simulink model "rear_differencial_dense_1"  (R2022b)
settings: Solver=FixedStepDiscrete  StartTime=0.0  StopTime=10.0  FixedStep=0.001  RelTol=1e-3  EnableMultiTasking=on
PreLoadFcn:
  | PowerOn_data
InitFcn:
  | EcoCoder_PreCheckLic();
values from neighbouring files (symbols this model uses):
  Accelerate_Percent_BreakPoints = uint8([0  2  5  10  20  30  40  50  60  70  80  90  100])    [PowerOn_data.m]
  MotorSpeed_BreakPoints = uint16(linspace(0,18000,13))    [PowerOn_data.m]
  Torque_Table = int8([ ... (first row only)    [PowerOn_data.m]
undefined symbols (not defined in the file or in its folder): HV_Botton, Inverter_Button, SC_Closed
libraries: CoderSF_BSW_Libs x83, SF_CanService_Libs x17, CoderSF_ADC2Volt_Libs x5, simulink x2, dspswit3 x1
(part 2 of 2)

== system rear_differencial_dense_1/CAN/CAN Read/SAS__CAN ==
  Bus Creator : BusCreator  Inputs=2
  Bus Creator1 : BusCreator  Inputs=7
  Read CAN Message : SF_CanService_Libs/Read CAN Message  typeCAN=Connected  channel=CAN_A  mEn=off  msgInfo=steering_angle_sensor  msgItermStore=Steering_Wheel_Angle  msgIterm=Steering_Wheel_Angle  valid=on  stale=on  motoBit=off  setSignalName=on  flgCustomMonitorVariableRules=on  defineSignalName=off  prefixSignal=''  flgValTest=off  flgNoFixed=on  tSample=Task_Inherit  modeCode=Parameterless
  Terminator : Terminator
  tag scope: SAS=global
  wires:
  Read CAN Message/7 -> Bus Creator1/5  "Function_SafetyRelated"
  Bus Creator1/1 -> [SAS]
  Read CAN Message/1 -> Bus Creator/1
  Read CAN Message/9 -> Bus Creator1/7  "SAS_SteeringAngle"
  Read CAN Message/6 -> Bus Creator1/4  "Not_Used"
  Read CAN Message/2 -> Bus Creator/2
  Read CAN Message/3 -> Bus Creator1/1  "SAS_CheckSum"
  Bus Creator/1 -> Terminator/1
  Read CAN Message/4 -> Bus Creator1/2  "Not_Used2"
  Read CAN Message/5 -> Bus Creator1/3  "SAS_MessageCounter"
  Read CAN Message/8 -> Bus Creator1/6  "SAS_SteeringAngle_Velocity"

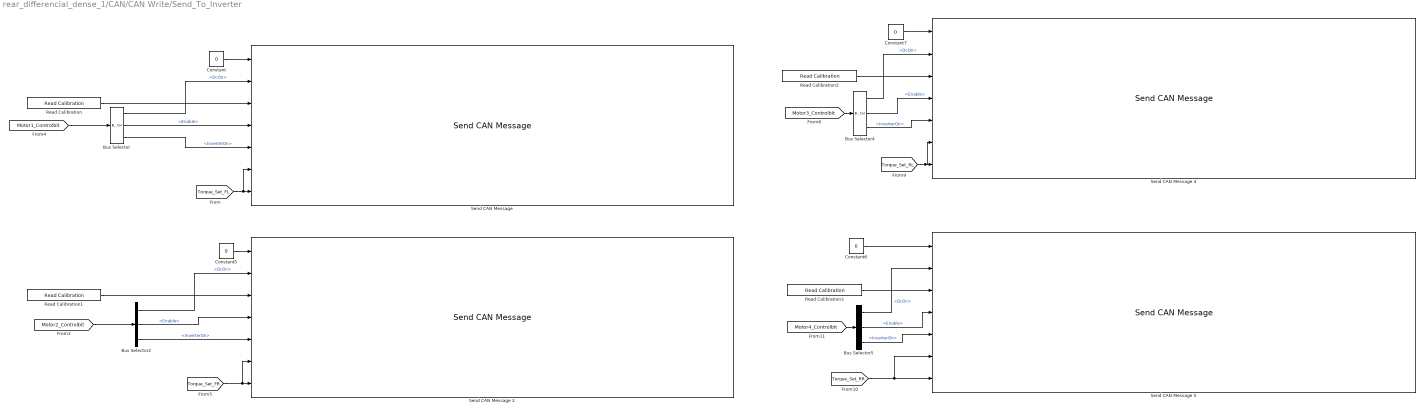
== system rear_differencial_dense_1/CAN/CAN Write/Send_To_Inverter ==
  Bus Selector{,2,4..5} (4 alike) : BusSelector  OutputSignals=DcOn,Enable,InverterOn
  Constant{,5..7} (4 alike) : Constant  Value=0  OutDataTypeStr=Inherit: Inherit via back propagation
  Read Calibration{,1..3} (4 alike) : CoderSF_BSW_Libs/Calibration & Measurement/Read Calibration  variable_name=errorset  variable_value=0  variable_type=boolean  variable_min=[]  variable_max=[]  unitStr=""  descStr=""
      settings: AttributesFormatString=value:%<variable_value> type:%<variable_type> max:%<variable_max> Min:%<variable_min>
  "Send CAN Message " : SF_CanService_Libs/Send CAN Message   typeCAN=Connected  channel=CAN_C  mEn=off  msgInfo=AMK_VCU_CAN_TorqueMode_factor_edited  msgItermStore=VCU1_0x184  msgIterm=VCU1_0x184  motoBit=off  flgNoFixed=on  tSample=Task_Inherit  modeCode=Parameterless  modeRound=Zero
  Send CAN Message 2 : SF_CanService_Libs/Send CAN Message   typeCAN=Connected  channel=CAN_C  mEn=off  msgInfo=AMK_VCU_CAN_TorqueMode_factor_edited  msgItermStore=VCU2_0x185  msgIterm=VCU2_0x185  motoBit=off  flgNoFixed=on  tSample=Task_Inherit  modeCode=Parameterless  modeRound=Zero
  Send CAN Message 4 : SF_CanService_Libs/Send CAN Message   typeCAN=Connected  channel=CAN_D  mEn=off  msgInfo=AMK_VCU_CAN_TorqueMode_factor_edited  msgItermStore=VCU3_0x188  msgIterm=VCU3_0x188  motoBit=off  flgNoFixed=on  tSample=Task_Inherit  modeCode=Parameterless  modeRound=Zero
  Send CAN Message 5 : SF_CanService_Libs/Send CAN Message   typeCAN=Connected  channel=CAN_D  mEn=off  msgInfo=AMK_VCU_CAN_TorqueMode_factor_edited  msgItermStore=VCU4_0x189  msgIterm=VCU4_0x189  motoBit=off  flgNoFixed=on  tSample=Task_Inherit  modeCode=Parameterless  modeRound=Zero
  wires:
  [Motor2_Controlbit] -> Bus Selector2/1
  Bus Selector4/2 -> Send CAN Message 4/4  "<Enable>"
  [Torque_Set_FL] -> "Send CAN Message "/6, "Send CAN Message "/7
  [Motor1_Controlbit] -> Bus Selector/1
  Read Calibration1/1 -> Send CAN Message 2/3
  Bus Selector/1 -> "Send CAN Message "/2  "<DcOn>"
  Bus Selector4/3 -> Send CAN Message 4/5  "<InverterOn>"
  [Motor3_Controlbit] -> Bus Selector4/1
  Bus Selector2/3 -> Send CAN Message 2/5  "<InverterOn>"
  Read Calibration2/1 -> Send CAN Message 4/3
  Bus Selector5/1 -> Send CAN Message 5/2  "<DcOn>"
  Bus Selector5/3 -> Send CAN Message 5/5  "<InverterOn>"
  Constant7/1 -> Send CAN Message 4/1
  [Motor4_Controlbit] -> Bus Selector5/1
  Constant5/1 -> Send CAN Message 2/1
  Bus Selector/2 -> "Send CAN Message "/4  "<Enable>"
  Read Calibration/1 -> "Send CAN Message "/3
  Bus Selector4/1 -> Send CAN Message 4/2  "<DcOn>"
  Constant/1 -> "Send CAN Message "/1
  Bus Selector5/2 -> Send CAN Message 5/4  "<Enable>"
  Read Calibration3/1 -> Send CAN Message 5/3
  Bus Selector2/1 -> Send CAN Message 2/2  "<DcOn>"
  [Torque_Set_FR] -> Send CAN Message 2/6, Send CAN Message 2/7
  Bus Selector/3 -> "Send CAN Message "/5  "<InverterOn>"
  [Torque_Set_RL] -> Send CAN Message 4/6, Send CAN Message 4/7
  Bus Selector2/2 -> Send CAN Message 2/4  "<Enable>"
  [Torque_Set_RR] -> Send CAN Message 5/6, Send CAN Message 5/7
  Constant6/1 -> Send CAN Message 5/1

== system rear_differencial_dense_1/CAN/CAN Write/Send_To_Recorder ==
  Bus Selector : BusSelector  OutputSignals=rxMCU_ActualTorque
  Bus Selector1 : BusSelector  OutputSignals=rxMCU_ActualTorque
  Bus Selector2 : BusSelector  OutputSignals=BatCurrent
  "Send CAN Message " : SF_CanService_Libs/Send CAN Message   typeCAN=Connected  channel=CAN_A  mEn=off  msgInfo=To_Recorder  msgItermStore=To_Recorder  msgIterm=To_Recorder  motoBit=off  flgNoFixed=on  tSample=Task_Inherit  modeCode=Parameterless  modeRound=Zero
  wires:
  [Motor3_Tag1] -> Bus Selector/1
  [Motor4_Tag1] -> Bus Selector1/1
  [BMS_INFO] -> Bus Selector2/1
  Bus Selector/1 -> "Send CAN Message "/2  "<rxMCU_ActualTorque>"
  Bus Selector1/1 -> "Send CAN Message "/1  "<rxMCU_ActualTorque>"
  Bus Selector2/1 -> "Send CAN Message "/3  "<BatCurrent>"

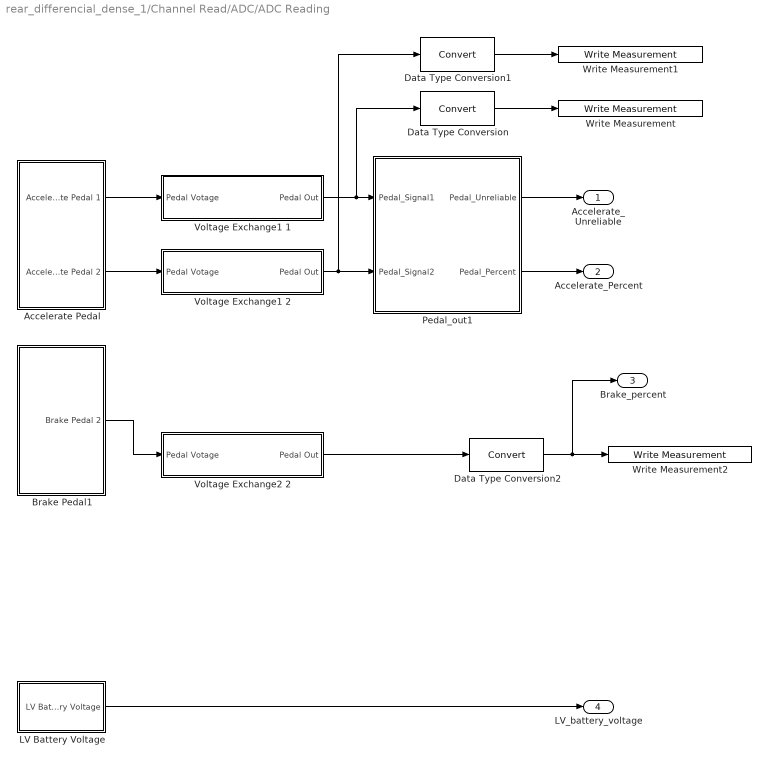
== system rear_differencial_dense_1/Channel Read/ADC/ADC Reading  ==
  Accelerate Pedal : Subsystem
  Brake Pedal1 : Subsystem
  Data Type Conversion : DataTypeConversion  SaturateOnIntegerOverflow=off  RndMeth=Floor
  Data Type Conversion1 : DataTypeConversion  SaturateOnIntegerOverflow=off  RndMeth=Floor
  Data Type Conversion2 : DataTypeConversion  SaturateOnIntegerOverflow=off  RndMeth=Floor
  LV Battery Voltage : Subsystem
  Pedal_out1 : Subsystem
  Voltage Exchange1 1 : Subsystem
  Voltage Exchange1 2 : Subsystem
  Voltage Exchange2 2 : Subsystem
  Write Measurement : CoderSF_BSW_Libs/Calibration & Measurement/Write Measurement  variable_name=ACC_per_h  variable_value=0  variable_type=single  numD=1  unitStr=""  descStr=""
      settings: AttributesFormatString=type:%<variable_type> Dimensions:%<numD>
  Write Measurement1 : CoderSF_BSW_Libs/Calibration & Measurement/Write Measurement  variable_name=ACC_per_l  variable_value=0  variable_type=single  numD=1  unitStr=""  descStr=""
      settings: AttributesFormatString=type:%<variable_type> Dimensions:%<numD>
  Write Measurement2 : CoderSF_BSW_Libs/Calibration & Measurement/Write Measurement  variable_name=brake_per_2  variable_value=0  variable_type=single  numD=1  unitStr=""  descStr=""
      settings: AttributesFormatString=type:%<variable_type> Dimensions:%<numD>
  Accelerate_Unreliable : Outport  VectorParamsAs1DForOutWhenUnconnected=off
  Accelerate_Percent : Outport  Port=2  VectorParamsAs1DForOutWhenUnconnected=off
  Brake_percent : Outport  Port=3
  LV_battery_voltage : Outport  Port=4  VectorParamsAs1DForOutWhenUnconnected=off
  wires:
  Accelerate Pedal/1(Accelerate Pedal 1) -> Voltage Exchange1 1/1(Pedal Votage)
  Accelerate Pedal/2(Accelerate Pedal 2) -> Voltage Exchange1 2/1(Pedal Votage)
  Brake Pedal1/1(Brake Pedal 2) -> Voltage Exchange2 2/1(Pedal Votage)
  Voltage Exchange1 1/1(Pedal Out) -> Data Type Conversion/1, Pedal_out1/1(Pedal_Signal1)
  Pedal_out1/1(Pedal_Unreliable) -> Accelerate_Unreliable/1
  Pedal_out1/2(Pedal_Percent) -> Accelerate_Percent/1
  Data Type Conversion/1 -> Write Measurement/1
  Voltage Exchange1 2/1(Pedal Out) -> Data Type Conversion1/1, Pedal_out1/2(Pedal_Signal2)
  Data Type Conversion1/1 -> Write Measurement1/1
  Voltage Exchange2 2/1(Pedal Out) -> Data Type Conversion2/1
  Data Type Conversion2/1 -> Brake_percent/1, Write Measurement2/1
  LV Battery Voltage/1(LV Battery Voltage) -> LV_battery_voltage/1

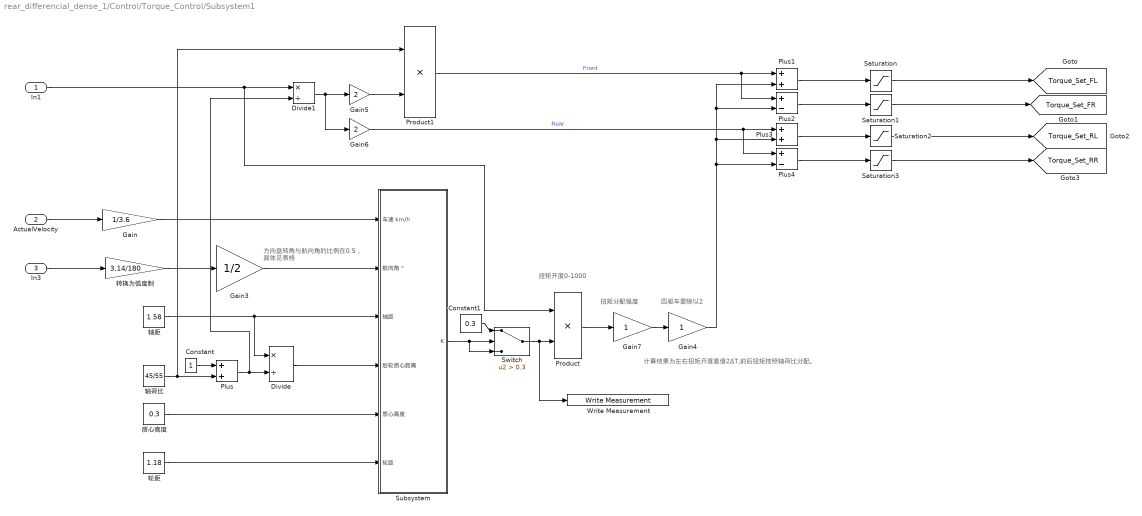
== system rear_differencial_dense_1/Control/Torque_Control/Subsystem1 ==
  note: 方向盘转角与航向角的比例在0.5，
      | 具体见表格
  note: 扭矩开度0-1000
  note: 四驱车要除以2
  note: 计算结果为左右扭矩开度差值2ΔT,前后扭矩按照轴荷比分配。
  note: 扭矩分配强度
  In1 : Inport
  ActualVelocity : Inport  Port=2
  In3 : Inport  Port=3
  Constant : Constant
  Constant1 : Constant  Value=0.3
  Divide : Product  Inputs=*/
  Divide1 : Product  Inputs=*/
  Gain : Gain  Gain=1/3.6
  Gain3 : Gain  Gain=1/2
  Gain4 : Gain
  Gain5 : Gain  Gain=2
  Gain6 : Gain  Gain=2
  Gain7 : Gain
  Plus : Sum
  Plus1 : Sum
  Plus2 : Sum  Inputs=+-
  Plus3 : Sum
  Plus4 : Sum  Inputs=+-
  Product : Product
  Product1 : Product
  Saturation : Saturate  UpperLimit=0  LowerLimit=0  OutDataTypeStr=uint16
  Saturation1 : Saturate  UpperLimit=750  LowerLimit=0  OutDataTypeStr=uint16
  Saturation2 : Saturate  UpperLimit=1000  LowerLimit=0  OutDataTypeStr=uint16
  Saturation3 : Saturate  UpperLimit=1000  LowerLimit=0  OutDataTypeStr=uint16
  Subsystem : Subsystem
  Switch : Switch  Criteria=u2 > Threshold  Threshold=0.3  OutDataTypeStr=single  SaturateOnIntegerOverflow=off  InputSameDT=off
  Write Measurement : CoderSF_BSW_Libs/Calibration & Measurement/Write Measurement  variable_name=differential_K  variable_value=0  variable_type=single  numD=1  unitStr=""  descStr=""
      settings: AttributesFormatString=type:%<variable_type> Dimensions:%<numD>
  质心高度 : Constant  Value=0.3
  转换为弧度制 : Gain  Gain=3.14/180
  轮距 : Constant  Value=1.18
  轴荷比 : Constant  Value=45/55
  轴距 : Constant  Value=1.58
  tag scope: Torque_Set_FL=global, Torque_Set_FR=global, Torque_Set_RL=global, Torque_Set_RR=global
  wires:
  In1/1 -> Product/1, Divide1/1
  轴荷比/1 -> Plus/2, Product1/1
  Saturation/1 -> [Torque_Set_FL]
  Constant/1 -> Plus/1
  轴距/1 -> Divide/1, Subsystem/3(轴距)
  Product1/1 -> Plus2/1, Plus1/1  "Front"
  Gain6/1 -> Plus4/1, Plus3/1  "Rear"
  Gain7/1 -> Gain4/1
  Gain4/1 -> Plus4/2, Plus3/2, Plus2/2, Plus1/2
  质心高度/1 -> Subsystem/5(质心高度)
  Product/1 -> Gain7/1
  Gain5/1 -> Product1/2
  Plus3/1 -> Saturation2/1
  Plus1/1 -> Saturation/1
  Plus2/1 -> Saturation1/1
  Plus4/1 -> Saturation3/1
  Divide1/1 -> Gain6/1, Gain5/1
  轮距/1 -> Subsystem/6(轮距)
  Gain3/1 -> Subsystem/2(航向角 °)
  Plus/1 -> Divide1/2, Divide/2
  Saturation1/1 -> [Torque_Set_FR]
  Saturation2/1 -> [Torque_Set_RL]
  Gain/1 -> Subsystem/1(车速 km/h)
  转换为弧度制/1 -> Gain3/1
  ActualVelocity/1 -> Gain/1
  In3/1 -> 转换为弧度制/1
  Divide/1 -> Subsystem/4(后轮质心距离)
  Subsystem/1(K) -> Switch/3, Switch/2
  Constant1/1 -> Switch/1
  Switch/1 -> Write Measurement/1, Product/2
  Saturation3/1 -> [Torque_Set_RR]

== system rear_differencial_dense_1/Channel Read/ADC/ADC Reading /Accelerate Pedal ==
  ADC Value To Volt : CoderSF_ADC2Volt_Libs/ADC Value To Volt  ResValue=12  RefValue=5  TypeOut=single  WithDiv=off  DivValue=0  SerValue=22
  ADC Value To Volt1 : CoderSF_ADC2Volt_Libs/ADC Value To Volt  ResValue=12  RefValue=5  TypeOut=single  WithDiv=off  DivValue=0  SerValue=22
  Read ADC Value : CoderSF_BSW_Libs/ADC/Read ADC Value  channel=1
  Read ADC Value1 : CoderSF_BSW_Libs/ADC/Read ADC Value  channel=2
  Write Measurement : CoderSF_BSW_Libs/Calibration & Measurement/Write Measurement  variable_name=ACC_Pedal_ADC1  variable_value=0  variable_type=single  numD=1  unitStr=""  descStr=""
      settings: AttributesFormatString=type:%<variable_type> Dimensions:%<numD>
  Write Measurement1 : CoderSF_BSW_Libs/Calibration & Measurement/Write Measurement  variable_name=ACC_Pedal_ADC2  variable_value=0  variable_type=single  numD=1  unitStr=""  descStr=""
      settings: AttributesFormatString=type:%<variable_type> Dimensions:%<numD>
  Accelerate Pedal 1 : Outport  VectorParamsAs1DForOutWhenUnconnected=off
  Accelerate Pedal 2 : Outport  Port=2  VectorParamsAs1DForOutWhenUnconnected=off
  wires:
  Read ADC Value1/1 -> ADC Value To Volt1/1
  ADC Value To Volt1/1 -> Write Measurement1/1, Accelerate Pedal 2/1
  Read ADC Value/1 -> ADC Value To Volt/1
  ADC Value To Volt/1 -> Write Measurement/1, Accelerate Pedal 1/1

== system rear_differencial_dense_1/Channel Read/ADC/ADC Reading /Brake Pedal1 ==
  ADC Value To Volt1 : CoderSF_ADC2Volt_Libs/ADC Value To Volt  ResValue=12  RefValue=5  TypeOut=single  WithDiv=off  DivValue=0  SerValue=22
  Data Type Conversion2 : DataTypeConversion  SaturateOnIntegerOverflow=off  RndMeth=Floor
  Read ADC Value1 : CoderSF_BSW_Libs/ADC/Read ADC Value  channel=5
  Write Measurement2 : CoderSF_BSW_Libs/Calibration & Measurement/Write Measurement  variable_name=brake_voltage__2  variable_value=0  variable_type=single  numD=1  unitStr=""  descStr=""
      settings: AttributesFormatString=type:%<variable_type> Dimensions:%<numD>
  Brake Pedal 2 : Outport  VectorParamsAs1DForOutWhenUnconnected=off
  wires:
  Read ADC Value1/1 -> ADC Value To Volt1/1
  ADC Value To Volt1/1 -> Data Type Conversion2/1, Brake Pedal 2/1
  Data Type Conversion2/1 -> Write Measurement2/1

== system rear_differencial_dense_1/Channel Read/ADC/ADC Reading /LV Battery Voltage ==
  ADC Value To Volt : CoderSF_ADC2Volt_Libs/ADC Value To Volt  ResValue=12  RefValue=32  TypeOut=uint8  WithDiv=on  DivValue=22  SerValue=3.48
  Read ADC Value : CoderSF_BSW_Libs/ADC/Read ADC Value  channel=17
  LV Battery Voltage : Outport  VectorParamsAs1DForOutWhenUnconnected=off
  wires:
  Read ADC Value/1 -> ADC Value To Volt/1
  ADC Value To Volt/1 -> LV Battery Voltage/1

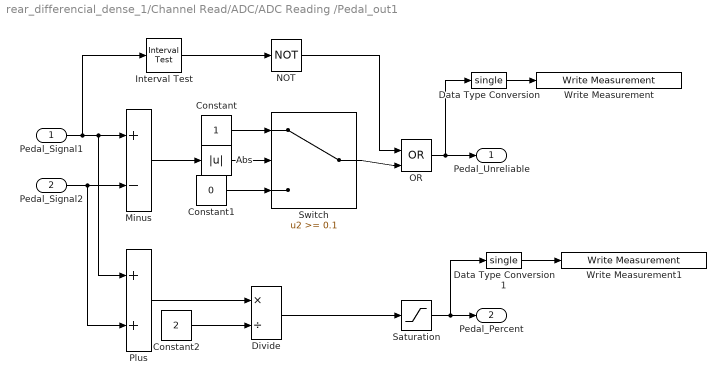
== system rear_differencial_dense_1/Channel Read/ADC/ADC Reading /Pedal_out1 ==
  Pedal_Signal1 : Inport
  Pedal_Signal2 : Inport  Port=2
  Abs : Abs  SaturateOnIntegerOverflow=off
  Constant : Constant  OutDataTypeStr=boolean
  Constant1 : Constant  Value=0  OutDataTypeStr=boolean
  Constant2 : Constant  Value=2
  Data Type Conversion : DataTypeConversion  OutDataTypeStr=single  SaturateOnIntegerOverflow=off  RndMeth=Floor
  Data Type Conversion1 : DataTypeConversion  OutDataTypeStr=single  SaturateOnIntegerOverflow=off  RndMeth=Floor
  Divide : Product  Inputs=*/
  Interval Test : simulink/Logic and Bit Operations/Interval Test  IntervalClosedRight=on  uplimit=1.05  IntervalClosedLeft=on  lowlimit=-0.05  OutDataTypeStr=boolean
  Minus : Sum  Inputs=+-
  NOT : Logic  Operator=NOT  IconShape=distinctive  AllPortsSameDT=off  OutDataTypeStr=boolean
  OR : Logic  Operator=OR  IconShape=distinctive  AllPortsSameDT=off  OutDataTypeStr=boolean
  Plus : Sum
  Saturation : Saturate  UpperLimit=1  LowerLimit=0  OutDataTypeStr=double
  Switch : Switch  Threshold=0.1  OutDataTypeStr=boolean  SaturateOnIntegerOverflow=off  InputSameDT=off
  Write Measurement : CoderSF_BSW_Libs/Calibration & Measurement/Write Measurement  variable_name=Pedal_Unreliable  variable_value=0  variable_type=single  numD=1  unitStr=""  descStr=""
      settings: AttributesFormatString=type:%<variable_type> Dimensions:%<numD>
  Write Measurement1 : CoderSF_BSW_Libs/Calibration & Measurement/Write Measurement  variable_name=Pedal_percent  variable_value=0  variable_type=single  numD=1  unitStr=""  descStr=""
      settings: AttributesFormatString=type:%<variable_type> Dimensions:%<numD>
  Pedal_Unreliable : Outport  VectorParamsAs1DForOutWhenUnconnected=off
  Pedal_Percent : Outport  Port=2  VectorParamsAs1DForOutWhenUnconnected=off
  wires:
  Pedal_Signal1/1 -> Interval Test/1, Plus/1, Minus/1
  Pedal_Signal2/1 -> Plus/2, Minus/2
  Abs/1 -> Switch/2
  Constant/1 -> Switch/1
  Constant1/1 -> Switch/3
  Plus/1 -> Divide/1
  Constant2/1 -> Divide/2
  Switch/1 -> OR/2
  OR/1 -> Data Type Conversion/1, Pedal_Unreliable/1
  Interval Test/1 -> NOT/1
  Divide/1 -> Saturation/1
  Saturation/1 -> Data Type Conversion1/1, Pedal_Percent/1
  NOT/1 -> OR/1
  Minus/1 -> Abs/1
  Data Type Conversion/1 -> Write Measurement/1
  Data Type Conversion1/1 -> Write Measurement1/1

== system rear_differencial_dense_1/Channel Read/ADC/ADC Reading /Voltage Exchange1 1 ==
  Pedal Votage : Inport
  Constant : Constant  Value=0.95
  Constant1 : Constant  Value=1.29
  Divide : Product  Inputs=*/
  Minus : Sum  Inputs=-+
  Pedal Out : Outport  VectorParamsAs1DForOutWhenUnconnected=off
  wires:
  Constant1/1 -> Divide/2
  Minus/1 -> Divide/1
  Divide/1 -> Pedal Out/1
  Constant/1 -> Minus/1
  Pedal Votage/1 -> Minus/2

== system rear_differencial_dense_1/Channel Read/ADC/ADC Reading /Voltage Exchange1 2 ==
  Pedal Votage : Inport
  Constant : Constant  Value=0.468
  Constant1 : Constant  Value=1.1
  Divide : Product  Inputs=*/
  Minus : Sum  Inputs=+-
  Pedal Out : Outport  VectorParamsAs1DForOutWhenUnconnected=off
  wires:
  Constant1/1 -> Divide/2
  Constant/1 -> Minus/2
  Minus/1 -> Divide/1
  Pedal Votage/1 -> Minus/1
  Divide/1 -> Pedal Out/1

== system rear_differencial_dense_1/Channel Read/ADC/ADC Reading /Voltage Exchange2 2 ==
  Pedal Votage : Inport
  Constant : Constant  Value=0.488
  Constant1 : Constant  Value=0.5
  Divide : Product  Inputs=*/
  Minus : Sum  Inputs=+-
  Pedal Out : Outport  VectorParamsAs1DForOutWhenUnconnected=off
  wires:
  Constant1/1 -> Divide/2
  Constant/1 -> Minus/2
  Minus/1 -> Divide/1
  Pedal Votage/1 -> Minus/1
  Divide/1 -> Pedal Out/1

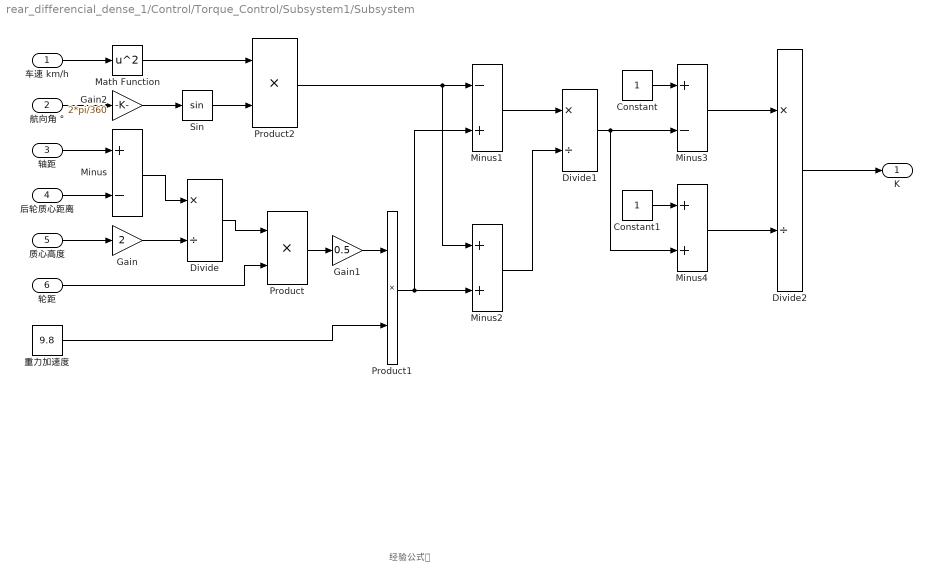
== system rear_differencial_dense_1/Control/Torque_Control/Subsystem1/Subsystem ==
  note: 经验公式👆
  车速 km/h : Inport
  航向角 ° : Inport  Port=2
  轴距 : Inport  Port=3
  后轮质心距离 : Inport  Port=4
  质心高度 : Inport  Port=5
  轮距 : Inport  Port=6
  Constant : Constant
  Constant1 : Constant
  Divide : Product  Inputs=*/
  Divide1 : Product  Inputs=*/
  Divide2 : Product  Inputs=*/
  Gain : Gain  Gain=2
  Gain1 : Gain  Gain=0.5
  Gain2 : Gain  Gain=2*pi/360  OutDataTypeStr=double
  Math Function : Math  Operator=square
  Minus : Sum  Inputs=+-
  Minus1 : Sum  Inputs=-+
  Minus2 : Sum
  Minus3 : Sum  Inputs=+-
  Minus4 : Sum
  Product : Product
  Product1 : Product
  Product2 : Product
  Sin : Trigonometry
  重力加速度 : Constant  Value=9.8
  K : Outport
  wires:
  轴距/1 -> Minus/1
  后轮质心距离/1 -> Minus/2
  质心高度/1 -> Gain/1
  Minus/1 -> Divide/1
  Gain/1 -> Divide/2
  轮距/1 -> Product/2
  Divide/1 -> Product/1
  Product/1 -> Gain1/1
  Gain1/1 -> Product1/1
  重力加速度/1 -> Product1/2
  Product1/1 -> Minus2/2, Minus1/2
  Math Function/1 -> Product2/1
  Sin/1 -> Product2/2
  Product2/1 -> Minus2/1, Minus1/1
  Minus2/1 -> Divide1/2
  Minus1/1 -> Divide1/1
  Divide1/1 -> Minus4/2, Minus3/2
  Constant/1 -> Minus3/1
  Constant1/1 -> Minus4/1
  Minus3/1 -> Divide2/1
  Minus4/1 -> Divide2/2
  Divide2/1 -> K/1
  Gain2/1 -> Sin/1
  车速 km/h/1 -> Math Function/1
  航向角 °/1 -> Gain2/1

== matlab function rear_differencial_dense_1/Control/Motor_Enable/MATLAB Function1 ==
  data: bSystemReady input; DcOn output; bDcOn input; bQuitDcOn input; bInverterOn input; bQuitInverterOn input; Inverter_Enable input; Enable output int16; InverterOn output int16; Ready output int16
function [DcOn, Enable, InverterOn, Ready]= Invertor( bSystemReady, bDcOn, bQuitDcOn, bInverterOn, bQuitInverterOn, Inverter_Enable)
DcOn       = int16(0);
Enable     = int16(0);
InverterOn = int16(0);
Ready      = int16(0);
if(Inverter_Enable == 1)
    if(bSystemReady    == 1)
        DcOn = int16(1);
        if(bDcOn == 1&&bQuitDcOn == 1)
            Enable     = int16(1);
            InverterOn = int16(1);
            if(bInverterOn == 1&&bQuitInverterOn == 1)
                Ready = int16(1);
            end
        end
    end
else
    DcOn = int16(1);
    Enable     = int16(0);
    InverterOn = int16(0);
    Ready = int16(0);
    if(bInverterOn == 1||bQuitInverterOn == 0)
        DcOn = int16(0);
    end
end

== matlab function rear_differencial_dense_1/Control/Motor_Enable/MATLAB Function ==
  data: bSystemReady input; DcOn output; bDcOn input; bQuitDcOn input; bInverterOn input; bQuitInverterOn input; Inverter_Enable input; Enable output int16; InverterOn output int16; Ready output int16
function [DcOn, Enable, InverterOn, Ready]= Invertor( bSystemReady, bDcOn, bQuitDcOn, bInverterOn, bQuitInverterOn, Inverter_Enable)
DcOn       = int16(0);
Enable     = int16(0);
InverterOn = int16(0);
Ready      = int16(0);
if(Inverter_Enable == 1)
    if(bSystemReady    == 1)
        DcOn = int16(1);
        if(bDcOn == 1&&bQuitDcOn == 1)
            Enable     = int16(1);
            InverterOn = int16(1);
            if(bInverterOn == 1&&bQuitInverterOn == 1)
                Ready = int16(1);
            end
        end
    end
else
    DcOn = int16(1);
    Enable     = int16(0);
    InverterOn = int16(0);
    Ready = int16(0);
    if(bInverterOn == 1||bQuitInverterOn == 0)
        DcOn = int16(0);
    end
end

== stateflow chart rear_differencial_dense_1/Control/StateMachine/Chart ==
  state LV
    Vehicle_Status=0;
  state HV
    Vehicle_Status=1;
  state DRIVE
    Vehicle_Status=2;
  (default) -> LV
  HV -> DRIVE [order 2] : [Invertor_Button==1&&SC_Closed==1 && Pedal_Unrelible==0]{Invertor_Enable=1;}
  LV -> HV : [HV_Button==1&&SC_Closed==1 && Pedal_Unrelible==0]{HV_Enable=1;}
  HV -> LV [order 1] : [SC_Closed==0]{HV_Enable=0;}
  DRIVE -> HV : [SC_Closed==0]{Invertor_Enable=0;}
  data: Vehicle_Status output; HV_Enable output; Invertor_Enable output; HV_Button input; Invertor_Button input; SC_Closed input; Pedal_Unrelible input

== matlab function rear_differencial_dense_1/Control/Motor_Enable/MATLAB Function2 ==
  data: bSystemReady input; DcOn output; bDcOn input; bQuitDcOn input; bInverterOn input; bQuitInverterOn input; Inverter_Enable input; Enable output int16; InverterOn output int16; Ready output int16
function [DcOn, Enable, InverterOn, Ready]= Invertor( bSystemReady, bDcOn, bQuitDcOn, bInverterOn, bQuitInverterOn, Inverter_Enable)
DcOn       = int16(0);
Enable     = int16(0);
InverterOn = int16(0);
Ready      = int16(0);
if(Inverter_Enable == 1)
    if(bSystemReady    == 1)
        DcOn = int16(1);
        if(bDcOn == 1&&bQuitDcOn == 1)
            Enable     = int16(1);
            InverterOn = int16(1);
            if(bInverterOn == 1&&bQuitInverterOn == 1)
                Ready = int16(1);
            end
        end
    end
else
    DcOn = int16(1);
    Enable     = int16(0);
    InverterOn = int16(0);
    Ready = int16(0);
    if(bInverterOn == 1||bQuitInverterOn == 0)
        DcOn = int16(0);
    end
end

== matlab function rear_differencial_dense_1/Control/Motor_Enable/MATLAB Function3 ==
  data: bSystemReady input; DcOn output; bDcOn input; bQuitDcOn input; bInverterOn input; bQuitInverterOn input; Inverter_Enable input; Enable output int16; InverterOn output int16; Ready output int16
function [DcOn, Enable, InverterOn, Ready]= Invertor( bSystemReady, bDcOn, bQuitDcOn, bInverterOn, bQuitInverterOn, Inverter_Enable)
DcOn       = int16(0);
Enable     = int16(0);
InverterOn = int16(0);
Ready      = int16(0);
if(Inverter_Enable == 1)
    if(bSystemReady    == 1)
        DcOn = int16(1);
        if(bDcOn == 1&&bQuitDcOn == 1)
            Enable     = int16(1);
            InverterOn = int16(1);
            if(bInverterOn == 1&&bQuitInverterOn == 1)
                Ready = int16(1);
            end
        end
    end
else
    DcOn = int16(1);
    Enable     = int16(0);
    InverterOn = int16(0);
    Ready = int16(0);
    if(bInverterOn == 1||bQuitInverterOn == 0)
        DcOn = int16(0);
    end
end
